simulink model "Modelo_LTI_Aumentado"  (R2026a)
settings: Solver=VariableStepAuto
values from neighbouring files (symbols this model uses):
  b_eq = b_m + b_l/(r_m2l^2)    (= 2.19444444444e-05)    [coeficientes.m]
  C_ts = 0.818    [coeficientes.m]
  J_eq = J_m + J_l/(r_m2l^2)    (= 4.58263888889e-05)    [coeficientes.m]
  L_d = 6.6e-3    (= 0.0066)    [coeficientes.m]
  L_q = 5.8e-3    (= 0.0058)    [coeficientes.m]
  lambda = 0.016    [coeficientes.m]
  Pp = 3    [coeficientes.m]
  R_tsamb = 146.7    [coeficientes.m]
undefined symbols (not defined in the file or in its folder): magnitude
settings Model: Creator=lamun  LastModifiedBy=lamun

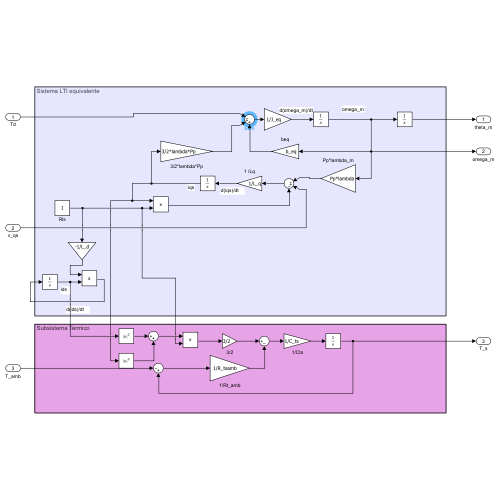
[thumbnail: Simulink's stored preview of the top-level diagram]
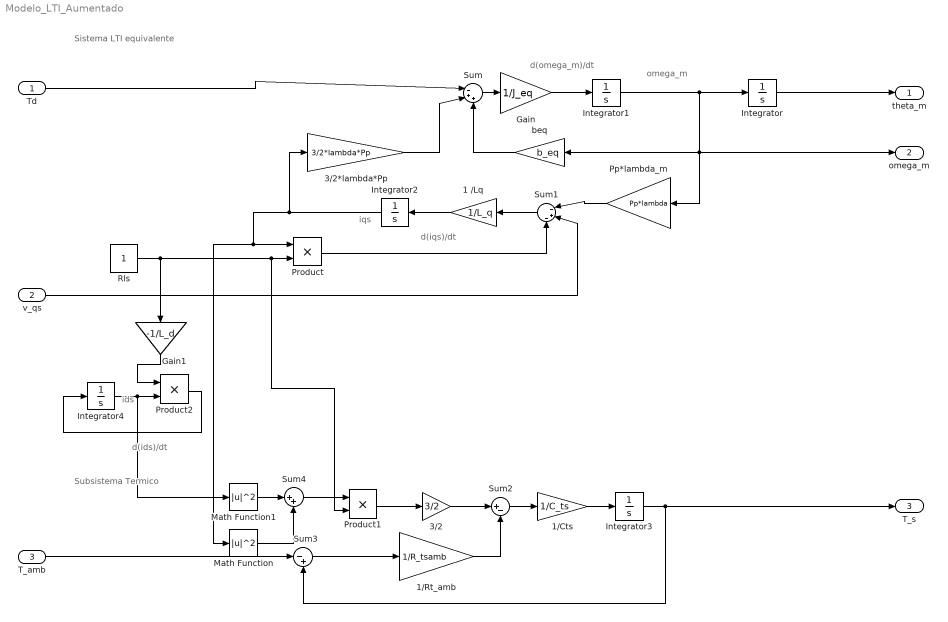
== system Modelo_LTI_Aumentado ==
  note: Sistema LTI equivalente
  note: Subsistema Termico
  note: omega_m
  note: d(omega_m)/dt
  note: d(iqs)/dt
  note: iqs
  note: d(ids)/dt
  note: ids
  Td : Inport
  v_qs : Inport  Port=2
  T_amb : Inport  Port=3
  1 /Lq : Gain  Gain=1/L_q
  1/Cts : Gain  Gain=1/C_ts
  1/Rt_amb : Gain  Gain=1/R_tsamb
  3/2 : Gain  Gain=3/2
  3/2*lambda*Pp : Gain  Gain=3/2*lambda*Pp
  Gain : Gain  Gain=1/J_eq
  Gain1 : Gain  Gain=-1/L_d
  Integrator{,1..4} (5 alike) : Integrator
  Math Function : Math  Operator=magnitude^2
  Math Function1 : Math  Operator=magnitude^2
  Pp*lambda_m : Gain  Gain=Pp*lambda
  Product : Product
  Product1 : Product
  Product2 : Product
  Rls : Constant
  Sum : Sum  Inputs=|-++
  Sum1 : Sum  Inputs=|-+-
  Sum2 : Sum  Inputs=|+-
  Sum3 : Sum  Inputs=|-+
  Sum4 : Sum  Inputs=|++
  beq : Gain  Gain=b_eq
  theta_m : Outport
  omega_m : Outport  Port=2
  T_s : Outport  Port=3
  wires:
  Sum/1 -> Gain/1
  Product1/1 -> 3/2/1
  T_amb/1 -> Sum3/1
  Sum3/1 -> 1/Rt_amb/1
  Product/1 -> Sum1/3
  Td/1 -> Sum/1
  3/2/1 -> Sum2/1
  Integrator1/1 -> Integrator/1, beq/1, omega_m/1, Pp*lambda_m/1
  Integrator2/1 -> 3/2*lambda*Pp/1, Product/1, Math Function/1
  Integrator3/1 -> T_s/1, Sum3/2
  Sum2/1 -> 1/Cts/1
  Sum1/1 -> 1 /Lq/1
  1 /Lq/1 -> Integrator2/1
  1/Rt_amb/1 -> Sum2/2
  1/Cts/1 -> Integrator3/1
  Gain/1 -> Integrator1/1
  3/2*lambda*Pp/1 -> Sum/2
  Integrator/1 -> theta_m/1
  v_qs/1 -> Sum1/2
  Pp*lambda_m/1 -> Sum1/1
  beq/1 -> Sum/3
  Product2/1 -> Integrator4/1
  Rls/1 -> Product1/2, Product/2, Gain1/1
  Integrator4/1 -> Math Function1/1, Product2/2
  Gain1/1 -> Product2/1
  Sum4/1 -> Product1/1
  Math Function/1 -> Sum4/2
  Math Function1/1 -> Sum4/1
